simulink model "sensorExpoler_encoder"  (R2026a)
settings: Solver=FixedStepAuto  StopTime=20  FixedStep=0.001
undefined symbols (not defined in the file or in its folder): Blocking, Non
libraries: amg_usbconverter_n_connect_lib x2, simulink x1
settings Model: Creator=pboon  LastModifiedBy=acer

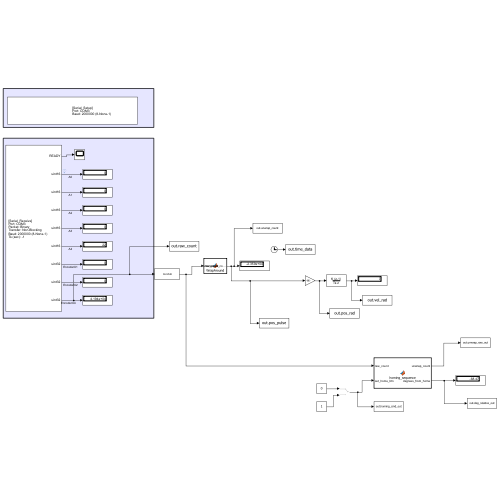
[thumbnail: Simulink's stored preview of the top-level diagram]
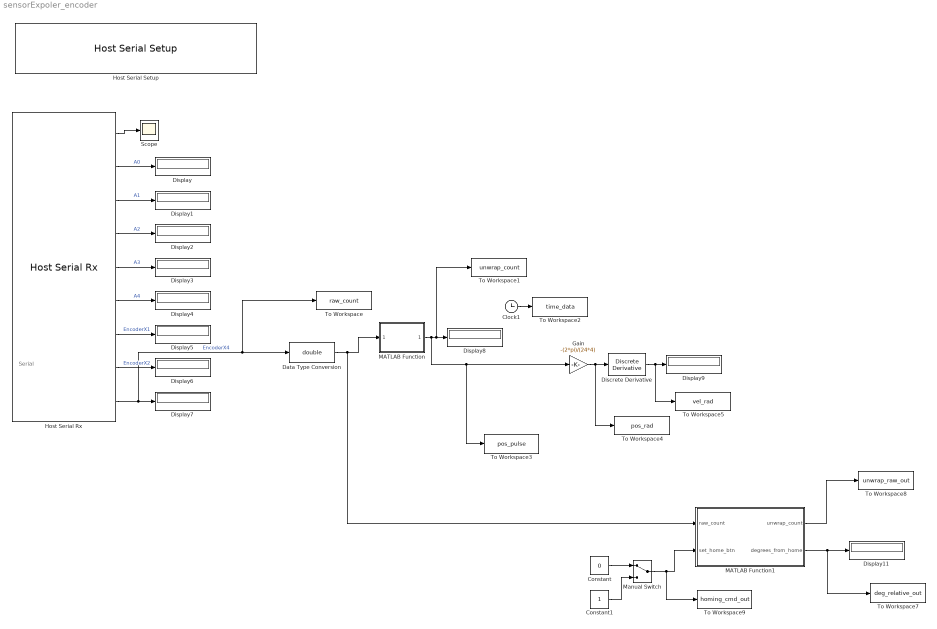
== system sensorExpoler_encoder ==
  note: Serial
  Clock1 : Clock
  Constant : Constant  Value=0
  Constant1 : Constant
  Data Type Conversion : DataTypeConversion  OutDataTypeStr=double  SaturateOnIntegerOverflow=off  RndMeth=Floor
  Discrete Derivative : simulink/Discrete/Discrete Derivative  gainval=1.0  ICPrevScaledInput=0.0  OutMin=[]  OutMax=[]  OutDataType=fixdt(1, 16)  OutScaling=2^-10  DoSatur=off
  Display{,1..9,11} (11 alike) : Display
  Gain : Gain  Gain=-(2*pi)/(24*4)
  Host Serial Rx : amg_usbconverter_n_connect_lib/Host Serial Rx  conf=rx  port=<auto>  baudrate=2000000  databits=8  parity=None  stopbit=1  flowcontrol=None  transfer=Non-Blocking  timeout=5  packetmode=Binary  enableinitialvalues=off  initialvalues=[]  binheader='25'  binterminator='4E 4E'  porttype_double=0  porttype_single=0  porttype_int8=0  porttype_uint8=0  porttype_int16=0  porttype_uint16=5  porttype_int32=0  porttype_uint32=3  asciiformat='%d,%f'  rx_asciiterminator="CRLF (0x0D 0x0A - \"\\r\\n\")"  tx_asciiterminator="CRLF (0x0D 0x0A - \"\\r\\n\")"  sampletime=0.001  enablecustomportlabel=off  cinputportlabel=0  coutputportlabel=A  portpinstr=0  blockid=HostSerialRx  inputporttype=[]  inputportwidth=[]  inputportlabel={}  outputporttype=[3 5 5 5 5 5 7 7 7]  outputportwidth=[1 1 1 1 1 1 1 1 1]  outputportlabel={'READY','uint16','uint16','uint16','uint16','uint16','uint32','uint32','uint32'}  compat=0  optionstring=[]  autoport='COM3'
  Host Serial Setup : amg_usbconverter_n_connect_lib/Host Serial Setup  conf=setup  port=<auto>  baudrate=2000000  databits=8  parity=None  stopbit=1  flowcontrol=None  transfer=Blocking  timeout=2  packetmode=Binary  initialvalues=[]  binheader='7E 7E'  binterminator='03 03'  porttype_double=0  porttype_single=1  porttype_int8=0  porttype_uint8=0  porttype_int16=0  porttype_uint16=0  porttype_int32=0  porttype_uint32=2  asciiformat='%d %u %x'  rx_asciiterminator="CRLF (0x0D 0x0A - \"\\r\\n\")"  tx_asciiterminator="CRLF (0x0D 0x0A - \"\\r\\n\")"  sampletime=-1  enablecustomportlabel=off  cinputportlabel=0  coutputportlabel=A  portpinstr=0  blockid=HostSerialSetup  inputporttype=[]  inputportwidth=[]  inputportlabel={}  outputporttype=[]  outputportwidth=[]  outputportlabel={}  compat=0  optionstring=[]  autoport='COM3'
  MATLAB Function : MATLAB Function  TreatAsAtomicUnit=on
  MATLAB Function1 : MATLAB Function  TreatAsAtomicUnit=on
  Manual Switch : ManualSwitch
  Scope : Scope
      settings: ActiveDisplayYMinimum=-0.12499999999999997  ActiveDisplayYMaximum=1.125
  To Workspace : ToWorkspace  VariableName=raw_count  SaveFormat=Timeseries  SampleTime=-1
  To Workspace1 : ToWorkspace  VariableName=unwrap_count  SaveFormat=Timeseries  SampleTime=-1
  To Workspace2 : ToWorkspace  VariableName=time_data  SaveFormat=Timeseries  SampleTime=-1
  To Workspace3 : ToWorkspace  VariableName=pos_pulse  SampleTime=-1
  To Workspace4 : ToWorkspace  VariableName=pos_rad  SampleTime=-1
  To Workspace5 : ToWorkspace  VariableName=vel_rad  SampleTime=-1
  To Workspace7 : ToWorkspace  VariableName=deg_relative_out  SampleTime=-1
  To Workspace8 : ToWorkspace  VariableName=unwrap_raw_out  SampleTime=-1
  To Workspace9 : ToWorkspace  VariableName=homing_cmd_out  SampleTime=-1
  wires:
  Host Serial Rx/2 -> Display/1  "A0"
  Host Serial Rx/3 -> Display1/1  "A1"
  Host Serial Rx/4 -> Display2/1  "A2"
  Host Serial Rx/5 -> Display3/1  "A3"
  Host Serial Rx/6 -> Display4/1  "A4"
  Host Serial Rx/7 -> Display5/1  "EncoderX1"
  Host Serial Rx/8 -> Display6/1  "EncoderX2"
  Host Serial Rx/9 -> To Workspace/1, Data Type Conversion/1, Display7/1  "EncoderX4"
  Host Serial Rx/1 -> Scope/1
  MATLAB Function/1(unwrapped_count) -> To Workspace3/1, Gain/1, To Workspace1/1, Display8/1
  Data Type Conversion/1 -> MATLAB Function/1(raw_count), MATLAB Function1/1(raw_count)
  Clock1/1 -> To Workspace2/1
  Gain/1 -> To Workspace4/1, Discrete Derivative/1
  Discrete Derivative/1 -> To Workspace5/1, Display9/1
  Manual Switch/1 -> To Workspace9/1, MATLAB Function1/2(set_home_btn)
  Constant/1 -> Manual Switch/1
  Constant1/1 -> Manual Switch/2
  MATLAB Function1/1(unwrap_count) -> To Workspace8/1
  MATLAB Function1/2(degrees_from_home) -> To Workspace7/1, Display11/1

== matlab function sensorExpoler_encoder/MATLAB Function ==
  data: raw_count input; unwrapped_count output
function unwrapped_count = WrapAround(raw_count)
    % กำหนดค่าคงที่ของระบบ
% เปลี่ยนค่าคงที่ให้ตรงกับ Hardware Timer (16-bit)
    PERIOD = 65535; 
    MAX_STEPS = 65536; 
    THRESHOLD = 32768; % ตั้งไว้ประมาณครึ่งหนึ่งของ MAX_STEPS

    % ใช้ persistent เพื่อให้ฟังก์ชันจดจำค่าในอดีตได้ในการรัน Loop รอบถัดไปของ Simulink
    persistent prev_raw;
    persistent accum_count;

    % กำหนดค่าเริ่มต้นเมื่อรันครั้งแรก
    if isempty(prev_raw)
        prev_raw = raw_count;
        accum_count = 0;
    end

    % 1. หาผลต่างระหว่างรอบปัจจุบันกับรอบที่แล้ว
    delta = raw_count - prev_raw;

    % 2. ตรวจสอบและชดเชยค่า Overflow / Underflow
    if delta < -THRESHOLD
        % กรณีหมุนเดินหน้า (เช่น 61439 -> 0) delta จะติดลบมาก (-61439)
        % ชดเชยโดยการบวก MAX_STEPS (-61439 + 61440 = +1)
        delta = delta + MAX_STEPS;
        
    elseif delta > THRESHOLD
        % กรณีหมุนถอยหลัง (เช่น 0 -> 61439) delta จะเป็นบวกมาก (+61439)
        % ชดเชยโดยการลบ MAX_STEPS (+61439 - 61440 = -1)
        delta = delta - MAX_STEPS;
    end

    % 3. นำ delta ที่ถูกต้องไปสะสมเป็น Total Count
    accum_count = accum_count + delta;
    
    % 4. อัปเดตค่าปัจจุบันไว้ใช้ในรอบหน้า
    prev_raw = raw_count;
    
    % 5. ส่งค่าที่ผ่านการแก้ Wrap-around ออกจาก Block
    unwrapped_count = accum_count;
end

== matlab function sensorExpoler_encoder/MATLAB Function1 ==
  data: raw_count input; unwrap_count output; set_home_btn input; degrees_from_home output
function [unwrap_count, degrees_from_home] = homing_sequence(raw_count, set_home_btn)
    persistent prev_raw unwrap_val home_offset;
    
    % ตั้งค่าเริ่มต้นเมื่อรันโปรแกรม
    if isempty(prev_raw)
        prev_raw = raw_count;
        unwrap_val = 0; 
        home_offset = 0; % ตัวแปรสำหรับจำจุด Home
    end
    
    % --- ส่วนที่ 1: จัดการ Wrap-around 16-bit ---
    delta = raw_count - prev_raw;
    if delta < -32768
        delta = delta + 65536;
    elseif delta > 32768
        delta = delta - 65536;
    end
    unwrap_val = unwrap_val + delta;
    prev_raw = raw_count;
    unwrap_count = unwrap_val; % ค่า Position รวมทั้งหมด
    
    % --- ส่วนที่ 2: Homing Sequence ---
    % ถ้ารับสัญญาณกดปุ่ม (set_home_btn = 1) ให้บันทึกตำแหน่งปัจจุบันเป็นจุด 0
    if set_home_btn == 1
        home_offset = unwrap_val;
    end
    
    % คำนวณระยะห่างจากจุด Home เป็น Pulses
    pulses_from_home = unwrap_val - home_offset;
    
    % --- ส่วนที่ 3: แปลงเป็นองศา ---
    % *** ต้องแก้ตัวเลข 8192 ให้ตรงกับฮาร์ดแวร์ที่ต่ออยู่ (เช่น AMT X4 = 8192, BOURNS X4 = 96) ***
    TOTAL_PULSES_PER_REV = 8192; 
    
    % กลับเครื่องหมายให้ทิศทางถูกต้อง
    degrees_from_home = -(pulses_from_home / TOTAL_PULSES_PER_REV) * 360;
end
